simulink model "techathonv5"  (R2024b)
settings: Solver=VariableStepAuto  StartTime=0.0  StopTime=10e-3  RelTol=1e-3
libraries: spsSeriesRLCBranchLib x7, spsVoltageMeasurementLib x7, spsCurrentMeasurementLib x2, spsACVoltageSourceLib x2, spsControlledVoltageSourceLib x1, spsGroundLib x1, spsDCVoltageSourceLib x1, sps_lib x1
settings Model: Creator=Yadnyesh  LastModifiedBy=Warad

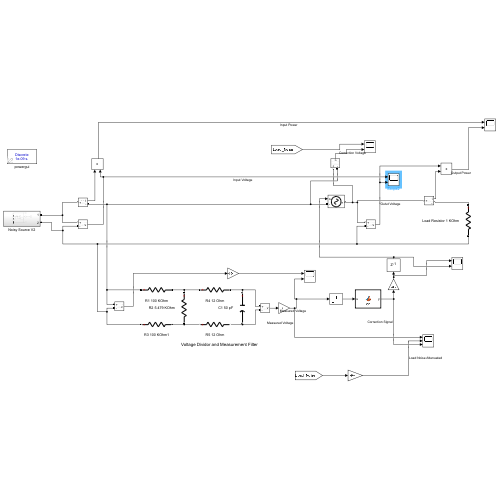
[thumbnail: Simulink's stored preview of the top-level diagram]
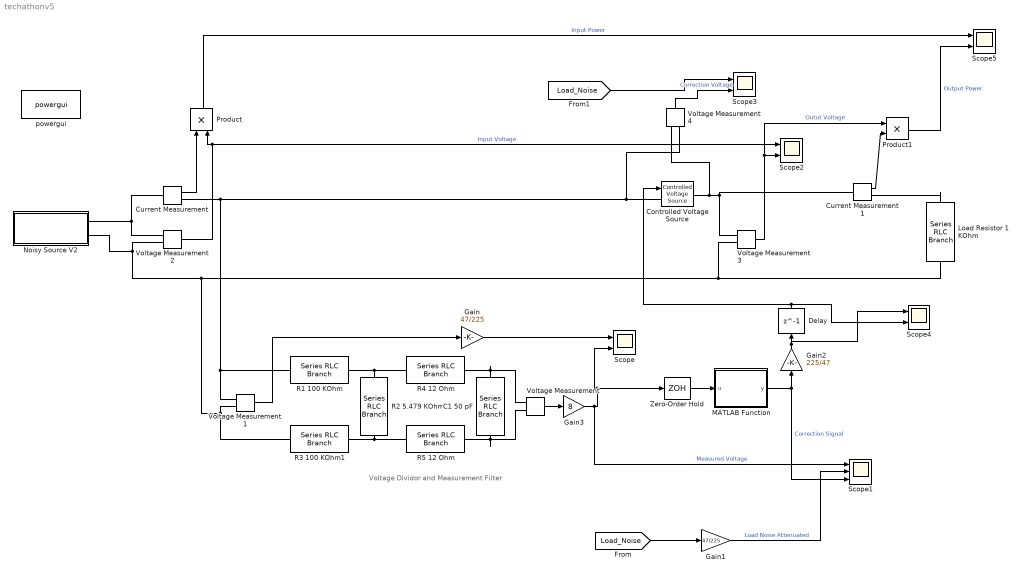
== system techathonv5 ==
  note: Voltage Dividor and Measurement Filter
  C1 50 pF : spsSeriesRLCBranchLib/Series RLC Branch  LConnTagsString=__new0  RConnTagsString=__new0  BranchType=C  Resistance=1  Inductance=1e-3  SetiL0=off  InitialCurrent=0  Capacitance=50e-12  Setx0=off  InitialVoltage=0  Measurements=None
  Controlled Voltage Source : spsControlledVoltageSourceLib/Controlled Voltage Source  Initialize=on  Source_Type=AC  Amplitude=0  Phase=0  Frequency=0  Measurements=None
  Current Measurement : spsCurrentMeasurementLib/Current Measurement  PhasorSimulation=off  OutputType=Complex  PSBequivalent=0
  Current Measurement1 : spsCurrentMeasurementLib/Current Measurement  PhasorSimulation=off  OutputType=Complex  PSBequivalent=0
  Delay : Delay  DelayLength=1  InputProcessing=Columns as channels (frame based)
  Gain : Gain  Gain=47/225
  Gain1 : Gain  Gain=47/225
  Gain2 : Gain  Gain=225/47
  Gain3 : Gain  Gain=8
  Load Resistor 1 KOhm : spsSeriesRLCBranchLib/Series RLC Branch  LConnTagsString=__new0  RConnTagsString=__new0  BranchType=R  Resistance=1e+3  Inductance=1e-3  SetiL0=off  InitialCurrent=0  Capacitance=1e-6  Setx0=off  InitialVoltage=0  Measurements=None
  MATLAB Function : MATLAB Function  TreatAsAtomicUnit=on
  Noisy Source V2 : Subsystem
  Product : Product
  Product1 : Product
  R1 100 KOhm : spsSeriesRLCBranchLib/Series RLC Branch  LConnTagsString=__new0  RConnTagsString=__new0  BranchType=R  Resistance=100e+3  Inductance=1e-3  SetiL0=off  InitialCurrent=0  Capacitance=1e-6  Setx0=off  InitialVoltage=0  Measurements=None
  R2 5.479 KOhm : spsSeriesRLCBranchLib/Series RLC Branch  LConnTagsString=__new0  RConnTagsString=__new0  BranchType=R  Resistance=5.479e+3  Inductance=1e-3  SetiL0=off  InitialCurrent=0  Capacitance=1e-6  Setx0=off  InitialVoltage=0  Measurements=None
  R3 100 KOhm1 : spsSeriesRLCBranchLib/Series RLC Branch  LConnTagsString=__new0  RConnTagsString=__new0  BranchType=R  Resistance=100e+3  Inductance=1e-3  SetiL0=off  InitialCurrent=0  Capacitance=1e-6  Setx0=off  InitialVoltage=0  Measurements=None
  R4 12 Ohm : spsSeriesRLCBranchLib/Series RLC Branch  LConnTagsString=__new0  RConnTagsString=__new0  BranchType=R  Resistance=12  Inductance=1e-3  SetiL0=off  InitialCurrent=0  Capacitance=1e-6  Setx0=off  InitialVoltage=0  Measurements=None
  R5 12 Ohm : spsSeriesRLCBranchLib/Series RLC Branch  LConnTagsString=__new0  RConnTagsString=__new0  BranchType=R  Resistance=12  Inductance=1e-3  SetiL0=off  InitialCurrent=0  Capacitance=1e-6  Setx0=off  InitialVoltage=0  Measurements=None
  Scope{,2..5} (5 alike) : Scope  NumInputPorts=2
  Scope1 : Scope  NumInputPorts=3
  Voltage Measurement{,1..4} (5 alike) : spsVoltageMeasurementLib/Voltage Measurement  PhasorSimulation=off  OutputType=Complex  PSBequivalent=0
  Zero-Order Hold : ZeroOrderHold  SampleTime=1/20000
  powergui : sps_lib/powergui  Priority=1  SimulationMode=Discrete  SampleTime=1e-9  frequency=60  Iterations=50  frequencyindice=0  Pbase=100e6  ErrMax=1e-4  UnitsV=kV  UnitsW=MW  buscounter=0  FunctionMessages=off  echomessages=off  EnableUseOfTLC=off  CurrentSourceSwitches=off  DisableSnubberDevices=off  DisableRonSwitches=off  DisableVfSwitches=off  DisplayEquations=off  AutomaticDiscreteSolvers=off  SolverType=Tustin/Backward Euler (TBE)  Interpol=off  ExternalGateDelay=off  methode=off  Ts=100  x0status=blocks  SPID=on  SwTol=0  HookPort=off  NonlinearTolerance=1e-4  nMaxIteration=100  ContinueOnMaxIteration=off  RestoreLinks=warning  ResistiveCurrentMeasurement=off  Frange=[0:2:500]  Ylog=off  Xlog=on  ShowGrid=off  save=off  variable=ZData  structure=0  ZoomFFT=off  StartTime=0.0  cycles=1  DisplayStyle=1  fundamental=60  FreqAxis=off  MaxFrequency=1000  frequencyindicesteady=1  RmsSteady=1  display=off
  wires:
  Voltage Measurement/1 -> Gain3/1
  Voltage Measurement1/1 -> Gain/1
  Gain/1 -> Scope/1
  [Load_Noise] -> Gain1/1
  Zero-Order Hold/1 -> MATLAB Function/1(u)
  Gain1/1 -> Scope1/2  "Load Noise Attenuated"
  Voltage Measurement2/1 -> Product/2, Scope2/1  "Input Voltage"
  Voltage Measurement3/1 -> Product1/1, Scope2/2  "Outut Voltage"
  Delay/1 -> Scope4/2, Controlled Voltage Source/1
  MATLAB Function/1(y) -> Scope1/3, Gain2/1  "Correction Signal"
  Gain2/1 -> Scope4/1, Delay/1
  Voltage Measurement4/1 -> Scope3/2  "Correction Voltage"
  [Load_Noise] -> Scope3/1
  Current Measurement/1 -> Product/1
  Current Measurement1/1 -> Product1/2
  Product/1 -> Scope5/1  "Input Power"
  Product1/1 -> Scope5/2  "Output Power"
  Gain3/1 -> Scope/2, Zero-Order Hold/1, Scope1/1  "Measured Voltage"
  connections:
  R1 100 KOhm/RConn1 -- R4 12 Ohm/LConn1 -- R2 5.479 KOhm/LConn1
  Voltage Measurement3/LConn2 -- Load Resistor 1 KOhm/RConn1 -- Voltage Measurement2/LConn2 -- Noisy Source V2/RConn2 -- R3 100 KOhm1/LConn1 -- Voltage Measurement1/LConn2
  Controlled Voltage Source/RConn1 -- Voltage Measurement3/LConn1 -- Current Measurement1/LConn1 -- Voltage Measurement4/LConn1
  Voltage Measurement2/LConn1 -- Current Measurement/LConn1 -- Noisy Source V2/RConn1
  R4 12 Ohm/RConn1 -- C1 50 pF/LConn1 -- Voltage Measurement/LConn1
  R5 12 Ohm/RConn1 -- C1 50 pF/RConn1 -- Voltage Measurement/LConn2
  Voltage Measurement4/LConn2 -- Current Measurement/RConn1 -- Voltage Measurement1/LConn1 -- R1 100 KOhm/LConn1 -- Controlled Voltage Source/LConn1
  Load Resistor 1 KOhm/LConn1 -- Current Measurement1/RConn1
  R5 12 Ohm/LConn1 -- R3 100 KOhm1/RConn1 -- R2 5.479 KOhm/RConn1

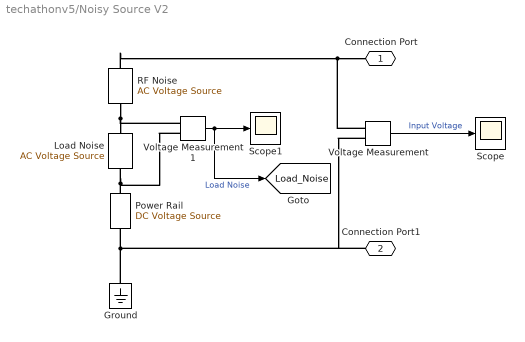
== system techathonv5/Noisy Source V2 ==
  Ground : spsGroundLib/Ground  LConnTagsString=a
  Load Noise : spsACVoltageSourceLib/AC Voltage Source  Amplitude=0.5  Phase=0  Frequency=500  SampleTime=1e-7  Measurements=None  BusType=swing  Pref=10e3  Qref=0  Qmin=-inf  Qmax=+inf
  Power Rail : spsDCVoltageSourceLib/DC Voltage Source  Amplitude=10.5  Measurements=None
  RF Noise : spsACVoltageSourceLib/AC Voltage Source  Amplitude=20e-3  Phase=0  Frequency=10e+6  SampleTime=1e-9  Measurements=None  BusType=swing  Pref=10e3  Qref=0  Qmin=-inf  Qmax=+inf
  Scope : Scope
  Scope1 : Scope
  Voltage Measurement : spsVoltageMeasurementLib/Voltage Measurement  PhasorSimulation=off  OutputType=Complex  PSBequivalent=0
  Voltage Measurement1 : spsVoltageMeasurementLib/Voltage Measurement  PhasorSimulation=off  OutputType=Complex  PSBequivalent=0
  Connection Port : PMIOPort  Side=Right
  Connection Port1 : PMIOPort  Port=2  Side=Right
  tag scope: Load_Noise=global
  wires:
  Voltage Measurement/1 -> Scope/1  "Input Voltage"
  Voltage Measurement1/1 -> Scope1/1, [Load_Noise]  "Load Noise"
  connections:
  Ground/LConn1 -- Voltage Measurement/LConn2 -- Connection Port1/RConn1 -- Power Rail/LConn1
  Power Rail/RConn1 -- Voltage Measurement1/LConn2 -- Load Noise/LConn1
  Voltage Measurement/LConn1 -- RF Noise/RConn1 -- Connection Port/RConn1
  RF Noise/LConn1 -- Voltage Measurement1/LConn1 -- Load Noise/RConn1

== matlab function techathonv5/MATLAB Function ==
  data: u input; y output
function y = fcn(u)
%% Discrete high-pass filter for DC + ripple separation
%% - Robust DC blocker (industry standard)
%% - Stable for large DC offsets
%% - Suitable for STM32 implementation

persistent u_prev y_prev initialized

if isempty(initialized)
    u_prev = u;
    y_prev = 0;
    initialized = true;
end

%% Parameters
fs = 200000;     % sample rate
fc = 50;        % cutoff (Hz)

alpha = exp(-2*pi*fc/fs);

%% DC blocking high-pass filter
y = (u - u_prev) + alpha * y_prev;

%% State update
u_prev = u;
y_prev = y;

%% Intentional inversion
y = -y;

%% Fail-safe
if ~isfinite(y)
    y = 0;
    u_prev = u;
    y_prev = 0;
end
